simulink model "Final_Sintonizacion_P_PI_PID"  (R2021a)
settings: Solver=VariableStepAuto  StartTime=0.0  StopTime=100  RelTol=1e-3
values from neighbouring files (symbols this model uses):
  q0 = (Q(2)-A(2)+1)/B(2)    [MatLab_Final.m]
  q1 = (Q(3)+A(2))/B(2)    [MatLab_Final.m]
libraries: cstblocks x1
settings Model: Creator=Pablo  LastModifiedBy=Pablo

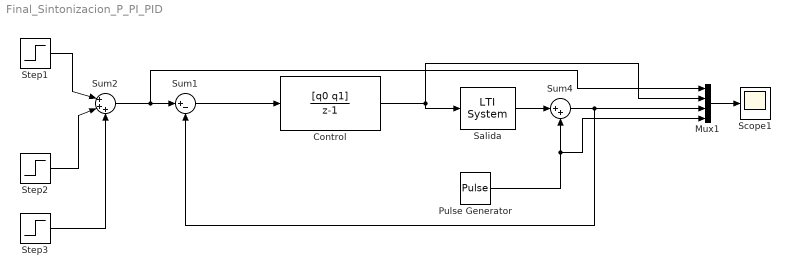
== system Final_Sintonizacion_P_PI_PID ==
  Control : DiscreteTransferFcn  Numerator=[q0 q1]  Denominator=[1 -1]
  Mux1 : Mux
  Pulse Generator : DiscretePulseGenerator  PulseType=Time based  Period=100  PulseWidth=50
  Salida : cstblocks/LTI System  sys=Gz  IC=[]
  Scope1 : Scope
  Step1 : Step  Time=0  After=10  SampleTime=0
  Step2 : Step  Time=31  After=30  SampleTime=0
  Step3 : Step  Time=61  After=-10  SampleTime=0
  Sum1 : Sum  Inputs=|+-
  Sum2 : Sum  Inputs=|+++
  Sum4 : Sum  Inputs=|++
  wires:
  Control/1 -> Salida/1, Mux1/2
  Sum1/1 -> Control/1
  Mux1/1 -> Scope1/1
  Step2/1 -> Sum2/2
  Step3/1 -> Sum2/3
  Step1/1 -> Sum2/1
  Sum2/1 -> Mux1/1, Sum1/1
  Salida/1 -> Sum4/1
  Pulse Generator/1 -> Mux1/4, Sum4/2
  Sum4/1 -> Mux1/3, Sum1/2
